simulink model "zoom_adc_single_pol"  (Simulink 7.8)
settings: Solver=FixedStepDiscrete  SolverMode=SingleTasking  StartTime=0.0  StopTime=4096  RelTol=1e-3
undefined symbols (not defined in the file): pfb_coeff_gen_calc
libraries: xbsIndex_r4 x413, casper_library_misc x48, xps_library x31, casper_library_delays x8, simulink x1
(part 1 of 6)
settings Model: Creator=jayanth  LastModifiedBy=dprice
settings Model: ModifiedComment=|
  | dprice -- Sun Apr 21 13:10:26 2013 -- Version 1.123
  | 
  | Added unsigned snap block to quant
settings Model: ModifiedHistory=|
  | dprice -- Sun Apr 21 13:10:26 2013 -- Version 1.123
  | 
  | Added unsigned snap block to quant
  | 
  | dprice -- Sun Apr 21 12:06:49 2013 -- Version 1.122
  | 
  | 
  | dprice -- Sun Apr 21 11:54:51 2013 -- Version 1.121
  | 
  | Changed over to quant block, added snap_quant for debugging
  | 
  | dprice -- Sun Apr 21 11:40:57 2013 -- Version 1.120
  | 
  | 
  | dprice -- Sun Apr 21 10:53:59 2013 -- Version 1.119
  | 
  | pkt_en going high now resets the packet counter in the header, and resets the 10 GbE core.
  | 
  | dprice -- Sat Apr 20 15:05:59 2013 -- Version 1.118
  | 
  | Fixed slice bug
  | 
  | dprice -- Sat Apr 20 14:12:55 2013 -- Version 1.117
  | 
  | Added a snap block after the quant
  | 
  | dprice -- Sat Apr 20 14:02:46 2013 -- Version 1.116
  | 
  | Trying to stop malformed packet being sent. Added in lots of pkt_en checks, so data is only valid when pkt_en is high
  | 
  | dprice -- Fri Apr 19 10:47:57 2013 -- Version 1.115
  | 
  | Switching to black boxed fft
settings DebuggingCC: FcnCallInpInsideContextMsg=Use local settings

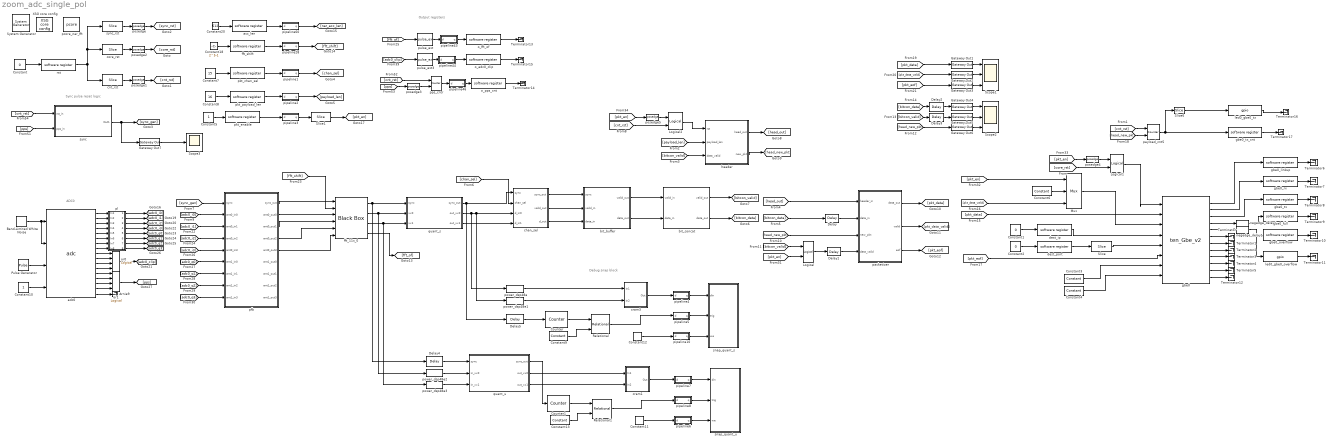
== system zoom_adc_single_pol ==
  note: Sync pulse reset logic
  note: ADC0
  note: Output registers
  note: Debug snap block
  " System Generator" : xbsIndex_r4/ System Generator  Tag=genX  xilinxfamily=virtex5  part=xc5vsx95t  speed=-1  package=ff1136  synthesis_tool=XST  clock_wrapper=Clock Enables  directory=./zoom_adc_single_pol/sysgen  proj_type=Project Navigator  Synth_file=XST Defaults  Impl_file=ISE Defaults  testbench=off  simulink_period=1  sysclk_period=5  dcm_input_clock_period=100  incr_netlist=off  trim_vbits=Everywhere in SubSystem  dbl_ovrd=According to Block Masks  core_generation=According to Block Masks  run_coregen=off  deprecated_control=off  eval_field=0  block_type=sysgen
  Arnie9 : Terminator
  Band-Limited White Noise : simulink/Sources/Band-Limited White Noise  Cov=[0.1]  Ts=0.1  seed=[23341]
  Constant : Constant  Value=0
  Constant1 : Constant  Value=0
  Constant10 : Constant
  Constant11 : xbsIndex_r4/Constant  const=1  gui_display_data_type=Boolean  arith_type=Boolean  n_bits=32  bin_pt=0  preci_type=Single  exp_width=8  frac_width=24  explicit_period=on  period=1  equ=P=C  opselect=C  inp2=PCIN>>17  opr=+  inp1=P  carry=CIN  dbl_ovrd=off  block_type=constant
  Constant12 : xbsIndex_r4/Constant  const=1  gui_display_data_type=Boolean  arith_type=Boolean  n_bits=32  bin_pt=0  preci_type=Single  exp_width=8  frac_width=24  explicit_period=on  period=1  equ=P=C  opselect=C  inp2=PCIN>>17  opr=+  inp1=P  carry=CIN  dbl_ovrd=off  block_type=constant
  Constant13 : xbsIndex_r4/Constant  const=0  gui_display_data_type=Fixed-point  arith_type=Signed (2's comp)  n_bits=3  bin_pt=0  preci_type=Single  exp_width=8  frac_width=24  explicit_period=on  period=1  equ=P=C  opselect=C  inp2=PCIN>>17  opr=+  inp1=P  carry=CIN  dbl_ovrd=off  block_type=constant
  Constant18 : Constant  Value=2^5-1
  Constant2 : Constant  Value=0
  Constant20 : Constant  Value=512
  Constant3 : xbsIndex_r4/Constant  const=1  gui_display_data_type=Boolean  arith_type=Boolean  n_bits=16  bin_pt=14  preci_type=Single  exp_width=8  frac_width=24  explicit_period=on  period=1  equ=P=C  opselect=C  inp2=PCIN>>17  opr=+  inp1=P  carry=CIN  dbl_ovrd=off  block_type=constant
  Constant4 : xbsIndex_r4/Constant  const=0  gui_display_data_type=Boolean  arith_type=Boolean  n_bits=16  bin_pt=14  preci_type=Single  exp_width=8  frac_width=24  explicit_period=on  period=1  equ=P=C  opselect=C  inp2=PCIN>>17  opr=+  inp1=P  carry=CIN  dbl_ovrd=off  block_type=constant
  Constant5 : Constant
  Constant6 : xbsIndex_r4/Constant  const=0  gui_display_data_type=Boolean  arith_type=Boolean  n_bits=16  bin_pt=14  preci_type=Single  exp_width=8  frac_width=24  explicit_period=off  period=1  equ=P=C  opselect=C  inp2=PCIN>>17  opr=+  inp1=P  carry=CIN  dbl_ovrd=off  block_type=constant
  Constant7 : Constant  Value=15
  Constant8 : Constant  Value=16
  Constant9 : xbsIndex_r4/Constant  const=0  gui_display_data_type=Fixed-point  arith_type=Signed (2's comp)  n_bits=3  bin_pt=0  preci_type=Single  exp_width=8  frac_width=24  explicit_period=on  period=1  equ=P=C  opselect=C  inp2=PCIN>>17  opr=+  inp1=P  carry=CIN  dbl_ovrd=off  block_type=constant
  Counter : xbsIndex_r4/Counter  cnt_type=Free Running  cnt_to=Inf  operation=Up  start_count=0  cnt_by_val=1  arith_type=Unsigned  n_bits=3  bin_pt=0  load_pin=off  rst=on  en=off  explicit_period=on  period=1  dbl_ovrd=off  use_behavioral_HDL=off  implementation=Fabric  block_type=counter
  Counter1 : xbsIndex_r4/Counter  cnt_type=Free Running  cnt_to=Inf  operation=Up  start_count=0  cnt_by_val=1  arith_type=Unsigned  n_bits=3  bin_pt=0  load_pin=off  rst=on  en=off  explicit_period=on  period=1  dbl_ovrd=off  use_behavioral_HDL=off  implementation=Fabric  block_type=counter
  Delay{,1..3} (4 alike) : xbsIndex_r4/Delay  rst=off  infoeditControl=Selection of Reset will increase slice count due to use of real FFs and instead of SRLs  en=off  latency=1  dbl_ovrd=off  reg_retiming=off  block_type=delay
  Delay4 : xbsIndex_r4/Delay  rst=off  infoeditControl=Selection of Reset will increase slice count due to use of real FFs and instead of SRLs  en=off  latency=4  dbl_ovrd=off  reg_retiming=off  block_type=delay
  Delay5 : xbsIndex_r4/Delay  rst=off  infoeditControl=Selection of Reset will increase slice count due to use of real FFs and instead of SRLs  en=off  latency=4  dbl_ovrd=off  reg_retiming=off  block_type=delay
  Gateway Out{1..7} (7 alike) : xbsIndex_r4/Gateway Out  inherit_from_input=off  hdl_port=on  timing_constraint=None  locs_specified=off  LOCs={}  UseAsDAC=off  DACChannel='1'  block_type=gatewayout
      settings: infoedit="Gateway out block.  Converts Xilinx fixed-point or floating-point type inputs into ouputs of type Simulink integer, single, double, or fixed point.<br><br>Hardware notes:  In hardware these blocks become top level output ports or are discarded, depending on how they are configured."
  Logical : xbsIndex_r4/Logical  logical_function=AND  inputs=2  en=off  latency=0  precision=Full  arith_type=Unsigned  n_bits=16  bin_pt=0  align_bp=on  dbl_ovrd=off  block_type=logical
  Logical1 : xbsIndex_r4/Logical  logical_function=OR  inputs=2  en=off  latency=0  precision=Full  arith_type=Unsigned  n_bits=16  bin_pt=0  align_bp=on  dbl_ovrd=off  block_type=logical
  Logical2 : xbsIndex_r4/Logical  logical_function=OR  inputs=2  en=off  latency=0  precision=Full  arith_type=Unsigned  n_bits=16  bin_pt=0  align_bp=on  dbl_ovrd=off  block_type=logical
  Mux : xbsIndex_r4/Mux  inputs=2  en=off  latency=0  precision=Full  arith_type=Unsigned  n_bits=16  bin_pt=14  quantization=Truncate  overflow=Wrap  dbl_ovrd=off  block_type=mux
  Pulse Generator : DiscretePulseGenerator  PulseType=Time based  Period=10  PulseWidth=5
  Relational : xbsIndex_r4/Relational  mode=a=b  en=off  latency=0  dbl_ovrd=off  block_type=relational
  Relational1 : xbsIndex_r4/Relational  mode=a=b  en=off  latency=0  dbl_ovrd=off  block_type=relational
  Scope1 : Scope  NumInputPorts=3
      settings: TimeRange=290.1459854014598  YMin=9.44473e+21~0~-1  YMax=3.5e+38~1~1
  Scope2 : Scope  NumInputPorts=3
      settings: TimeRange=290.1459854014598  YMin=0~0~0  YMax=1.2e+18~1~1
  Scope3 : Scope
      settings: SaveName=ScopeData6
  Slice : xbsIndex_r4/Slice  nbits=16  boolean_output=off  mode=Lower Bit Location + Width  bit1=0  base1=MSB of Input  bit0=0  base0=LSB of Input  dbl_ovrd=off  block_type=slice
  Slice1 : xbsIndex_r4/Slice  nbits=1  boolean_output=on  mode=Lower Bit Location + Width  bit1=1  base1=MSB of Input  bit0=0  base0=LSB of Input  dbl_ovrd=off  block_type=slice
      settings: block_version=10.1.3
  Slice6 : xbsIndex_r4/Slice  nbits=1  boolean_output=on  mode=Lower Bit Location + Width  bit1=0  base1=MSB of Input  bit0=15  base0=LSB of Input  dbl_ovrd=off  block_type=slice
      settings: block_version=10.1.3
  Terminator{,1..17} (18 alike) : Terminator
  XSG core config : xps_library/XSG core config  Tag=xps:xsg  hw_sys=ROACH:sx95t  ibob_linux=off  clk_src=adc0_clk  iBOB_clk_src=sys_clk  BEE2_ctrl_clk_src=sys_clk  BEE2_usr_clk_src=sys_clk  ROACH_clk_src=adc0_clk  ROACH2_clk_src=adc0_clk  CORR_clk_src=sys_clk  gpio_clk_io_group=iBOB:sma  gpio_clk_bit_index=0  clk_rate=200  sample_period=1  synthesis_tool=XST  mpc_type=powerpc440_ext
  acc_len : xps_library/software register  Tag=xps:sw_reg  io_dir=From Processor  arith_type=Unsigned  bitwidth=32  bin_pt=0  sample_period=1  gw_name=zoom_adc_single_pol_acc_len_user_data_out
      link override coarse_r01_acc_len_user_data_out: arith_type=Unsigned  n_bits=32  bin_pt=0  period=1
      link override coarse_r02_acc_len_user_data_out: arith_type=Unsigned  n_bits=32  bin_pt=0  period=1
      link override coarse_r03_acc_len_user_data_out: arith_type=Unsigned  n_bits=32  bin_pt=0  period=1
      link override coarse_r04_acc_len_user_data_out: arith_type=Unsigned  n_bits=32  bin_pt=0  period=1
      link override coarse_r06_acc_len_user_data_out: arith_type=Unsigned  n_bits=32  bin_pt=0  period=1
      link override coarse_r07_acc_len_user_data_out: arith_type=Unsigned  n_bits=32  bin_pt=0  period=1
      link override coarse_r08_acc_len_user_data_out: arith_type=Unsigned  n_bits=32  bin_pt=0  period=1
      link override coarse_r09_acc_len_user_data_out: arith_type=Unsigned  n_bits=32  bin_pt=0  period=1
      link override coarse_r10_acc_len_user_data_out: arith_type=Unsigned  n_bits=32  bin_pt=0  period=1
      link override coarse_r12_acc_len_user_data_out: arith_type=Unsigned  n_bits=32  bin_pt=0  period=1
      link override convert: arith_type=Unsigned  n_bits=32  bin_pt=0
      link override qdr_single_r01_acc_len_coarse_user_data_out: arith_type=Unsigned  n_bits=32  bin_pt=0  period=1
      link override qdr_single_r02_acc_len_coarse_user_data_out: arith_type=Unsigned  n_bits=32  bin_pt=0  period=1
      link override qdr_single_r04_acc_len_coarse_user_data_out: arith_type=Unsigned  n_bits=32  bin_pt=0  period=1
      link override r_spec_2048_r102_acc_len_user_data_out: arith_type=Unsigned  n_bits=32  bin_pt=0  period=1
      link override r_spec_2048_r102_nosim_acc_len_user_data_out: arith_type=Unsigned  n_bits=32  bin_pt=0  period=1
      link override r_spec_2048_r103_acc_len_user_data_out: arith_type=Unsigned  n_bits=32  bin_pt=0  period=1
      link override r_spec_2048_r104_acc_len_user_data_out: arith_type=Unsigned  n_bits=32  bin_pt=0  period=1
      link override r_spec_2048_r104_test0_acc_len_user_data_out: arith_type=Unsigned  n_bits=32  bin_pt=0  period=1
      link override r_spec_2048_r104_test_acc_len_user_data_out: arith_type=Unsigned  n_bits=32  bin_pt=0  period=1
      link override r_spec_2048_r105_acc_len_user_data_out: arith_type=Unsigned  n_bits=32  bin_pt=0  period=1
      link override r_spec_test0_acc_len_user_data_out: arith_type=Unsigned  n_bits=32  bin_pt=0  period=1
      link override r_spec_test4_acc_len_user_data_out: arith_type=Unsigned  n_bits=32  bin_pt=0  period=1
      link override roach_spec_acc_len_user_data_out: arith_type=Unsigned  n_bits=32  bin_pt=0  period=1
      link override roach_spec_no10gbe_acc_len_user_data_out: arith_type=Unsigned  n_bits=32  bin_pt=0  period=1
      link override roach_spec_rst_sync_cnt_user_data_out: arith_type=Unsigned  n_bits=32  bin_pt=0  period=1
      link override toast_256ch_16bit_r02_acc_len_user_data_out: arith_type=Unsigned  n_bits=32  bin_pt=0  period=1
      link override toast_256ch_16bit_r04_acc_len_user_data_out: arith_type=Unsigned  n_bits=32  bin_pt=0  period=1
      link override toast_256ch_16bit_r05_acc_len_user_data_out: arith_type=Unsigned  n_bits=32  bin_pt=0  period=1
  adc0 : xps_library/adc  Tag=xps:adc  adc_brd=adc0  adc_clk_rate=800  adc_interleave=off  sample_period=1
  bit_buffer : Subsystem
  bit_concat : Subsystem
  chan_sel : Subsystem
  cnt_rst : xbsIndex_r4/Slice  nbits=1  boolean_output=on  mode=Lower Bit Location + Width  bit1=0  base1=MSB of Input  bit0=0  base0=LSB of Input  dbl_ovrd=off  block_type=slice
  core_rst : xbsIndex_r4/Slice  nbits=1  boolean_output=on  mode=Lower Bit Location + Width  bit1=0  base1=MSB of Input  bit0=1  base0=LSB of Input  dbl_ovrd=off  block_type=slice
  cram1 : Subsystem  AncestorBlock=gavrt_library/cram  mask(cram){num_slice=2}
      mask prompts: num_slice "Number of slices"
      mask help: Concatenates inputs together after forcing binary point to zero.
      mask init:
      | cram_init(gcb, ...
      |     'num_slice', num_slice);
  cram3 : Subsystem  AncestorBlock=gavrt_library/cram  mask(cram){num_slice=2}
      mask prompts: num_slice "Number of slices"
      mask help: Concatenates inputs together after forcing binary point to zero.
      mask init:
      | cram_init(gcb, ...
      |     'num_slice', num_slice);
  dest_ip : xps_library/software register  Tag=xps:sw_reg  io_dir=From Processor  arith_type=Unsigned  bitwidth=32  bin_pt=0  sample_period=1  gw_name=zoom_adc_single_pol_dest_ip_user_data_out
      link override hipsr_tgbe3_dest_ip_user_data_out: arith_type=Unsigned  n_bits=32  bin_pt=0  period=1
  dest_port : xps_library/software register  Tag=xps:sw_reg  io_dir=From Processor  arith_type=Unsigned  bitwidth=32  bin_pt=0  sample_period=1  gw_name=zoom_adc_single_pol_dest_port_user_data_out
      link override hipsr_tgbe3_dest_port_user_data_out: arith_type=Unsigned  n_bits=32  bin_pt=0  period=1
  fft_11x_0 : xbsIndex_r4/Black Box  init_code=fft_32pt_11x_core_config  sim_method=Inactive  verbose=off  block_type=blackbox2
  fft_shift : xps_library/software register  Tag=xps:sw_reg  io_dir=From Processor  arith_type=Unsigned  bitwidth=32  bin_pt=0  sample_period=1  gw_name=zoom_adc_single_pol_fft_shift_user_data_out
      link override coarse_r01_acc_len_user_data_out: arith_type=Unsigned  n_bits=32  bin_pt=0  period=1
      link override coarse_r02_acc_len_user_data_out: arith_type=Unsigned  n_bits=32  bin_pt=0  period=1
      link override coarse_r03_acc_len_user_data_out: arith_type=Unsigned  n_bits=32  bin_pt=0  period=1
      link override coarse_r04_acc_len_user_data_out: arith_type=Unsigned  n_bits=32  bin_pt=0  period=1
      link override coarse_r06_acc_len_user_data_out: arith_type=Unsigned  n_bits=32  bin_pt=0  period=1
      link override coarse_r07_acc_len_user_data_out: arith_type=Unsigned  n_bits=32  bin_pt=0  period=1
      link override coarse_r08_acc_len_user_data_out: arith_type=Unsigned  n_bits=32  bin_pt=0  period=1
      link override coarse_r09_acc_len_user_data_out: arith_type=Unsigned  n_bits=32  bin_pt=0  period=1
      link override coarse_r10_acc_len_user_data_out: arith_type=Unsigned  n_bits=32  bin_pt=0  period=1
      link override coarse_r12_acc_len_user_data_out: arith_type=Unsigned  n_bits=32  bin_pt=0  period=1
      link override convert: arith_type=Unsigned  n_bits=32  bin_pt=0
      link override qdr_single_r01_acc_len_coarse_user_data_out: arith_type=Unsigned  n_bits=32  bin_pt=0  period=1
      link override qdr_single_r02_acc_len_coarse_user_data_out: arith_type=Unsigned  n_bits=32  bin_pt=0  period=1
      link override qdr_single_r04_acc_len_coarse_user_data_out: arith_type=Unsigned  n_bits=32  bin_pt=0  period=1
      link override r_spec_2048_r102_acc_len_user_data_out: arith_type=Unsigned  n_bits=32  bin_pt=0  period=1
      link override r_spec_2048_r102_nosim_acc_len_user_data_out: arith_type=Unsigned  n_bits=32  bin_pt=0  period=1
      link override r_spec_2048_r103_acc_len_user_data_out: arith_type=Unsigned  n_bits=32  bin_pt=0  period=1
      link override r_spec_2048_r104_acc_len_user_data_out: arith_type=Unsigned  n_bits=32  bin_pt=0  period=1
      link override r_spec_2048_r104_test0_acc_len_user_data_out: arith_type=Unsigned  n_bits=32  bin_pt=0  period=1
      link override r_spec_2048_r104_test_acc_len_user_data_out: arith_type=Unsigned  n_bits=32  bin_pt=0  period=1
      link override r_spec_2048_r105_acc_len_user_data_out: arith_type=Unsigned  n_bits=32  bin_pt=0  period=1
      link override r_spec_test0_acc_len_user_data_out: arith_type=Unsigned  n_bits=32  bin_pt=0  period=1
      link override r_spec_test4_acc_len_user_data_out: arith_type=Unsigned  n_bits=32  bin_pt=0  period=1
      link override roach_spec_acc_len_user_data_out: arith_type=Unsigned  n_bits=32  bin_pt=0  period=1
      link override roach_spec_no10gbe_acc_len_user_data_out: arith_type=Unsigned  n_bits=32  bin_pt=0  period=1
      link override roach_spec_rst_sync_cnt_user_data_out: arith_type=Unsigned  n_bits=32  bin_pt=0  period=1
      link override toast_256ch_16bit_r02_acc_len_user_data_out: arith_type=Unsigned  n_bits=32  bin_pt=0  period=1
      link override toast_256ch_16bit_r04_acc_len_user_data_out: arith_type=Unsigned  n_bits=32  bin_pt=0  period=1
      link override toast_256ch_16bit_r05_acc_len_user_data_out: arith_type=Unsigned  n_bits=32  bin_pt=0  period=1
  gbe0 : xps_library/ten_Gbe_v2  Tag=xps:tengbe_v2  port=0  rx_dist_ram=off  large_frames=on  show_param=off  pre_emph=3  swing=800  fab_en=on  fab_mac=hex2dec('123456780000')  fab_ip=192*(2^24) + 168*(2^16) + 5*(2^8) + 20*(2^0)  fab_udp=10000  fab_gate=1  cpu_rx_en=on  cpu_tx_en=on
  gbe0_full : xps_library/software register  Tag=xps:sw_reg  io_dir=To Processor  arith_type=Unsigned  bitwidth=32  bin_pt=0  sample_period=1  gw_name=zoom_adc_single_pol_gbe0_full_user_data_in
      link override convert: arith_type=Unsigned  n_bits=32  bin_pt=0
  gbe0_linkup : xps_library/software register  Tag=xps:sw_reg  io_dir=To Processor  arith_type=Unsigned  bitwidth=32  bin_pt=0  sample_period=1  gw_name=zoom_adc_single_pol_gbe0_linkup_user_data_in
      link override convert: arith_type=Unsigned  n_bits=32  bin_pt=0
  gbe0_overflow : xps_library/software register  Tag=xps:sw_reg  io_dir=To Processor  arith_type=Unsigned  bitwidth=32  bin_pt=0  sample_period=1  gw_name=zoom_adc_single_pol_gbe0_overflow_user_data_in
      link override convert: arith_type=Unsigned  n_bits=32  bin_pt=0
  gbe0_rx : xps_library/software register  Tag=xps:sw_reg  io_dir=To Processor  arith_type=Unsigned  bitwidth=32  bin_pt=0  sample_period=1  gw_name=zoom_adc_single_pol_gbe0_rx_user_data_in
      link override convert: arith_type=Unsigned  n_bits=32  bin_pt=0
  gbe0_tx : xps_library/software register  Tag=xps:sw_reg  io_dir=To Processor  arith_type=Unsigned  bitwidth=32  bin_pt=0  sample_period=1  gw_name=zoom_adc_single_pol_gbe0_tx_user_data_in
      link override convert: arith_type=Unsigned  n_bits=32  bin_pt=0
  gbe0_tx_cnt : xps_library/software register  Tag=xps:sw_reg  io_dir=To Processor  arith_type=Unsigned  bitwidth=32  bin_pt=0  sample_period=1  gw_name=zoom_adc_single_pol_gbe0_tx_cnt_user_data_in
      link override convert: arith_type=Unsigned  n_bits=32  bin_pt=0
  header : Subsystem
  led0_gbe0_overflow : xps_library/gpio  Tag=xps:gpio  io_group=ROACH:led  io_dir=out  arith_type=Boolean  bitwidth=1  bin_pt=0  bit_index=1  sample_period=1  use_single_ended=off  use_ddr=off  reg_iob=on  reg_clk_phase=0  termination=None
      link override convert: arith_type=Boolean  n_bits=1  bin_pt=0
  led0_gbe0_tx : xps_library/gpio  Tag=xps:gpio  io_group=ROACH:led  io_dir=out  arith_type=Boolean  bitwidth=1  bin_pt=0  bit_index=0  sample_period=1  use_single_ended=off  use_ddr=off  reg_iob=off  reg_clk_phase=0  termination=None
      link override convert: arith_type=Boolean  n_bits=1  bin_pt=0
  negedge_delay : casper_library_misc/negedge_delay  pulse_len=2^20
  negedge_delay1 : casper_library_misc/negedge_delay  pulse_len=2^20
  o_adc0_clip : xps_library/software register  Tag=xps:sw_reg  io_dir=To Processor  arith_type=Unsigned  bitwidth=32  bin_pt=0  sample_period=1  gw_name=zoom_adc_single_pol_o_adc0_clip_user_data_in
      link override convert: arith_type=Unsigned  n_bits=32  bin_pt=0
  o_fft_of : xps_library/software register  Tag=xps:sw_reg  io_dir=To Processor  arith_type=Unsigned  bitwidth=32  bin_pt=0  sample_period=1  gw_name=zoom_adc_single_pol_o_fft_of_user_data_in
      link override convert: arith_type=Unsigned  n_bits=32  bin_pt=0
  o_pps_cnt : xps_library/software register  Tag=xps:sw_reg  io_dir=To Processor  arith_type=Unsigned  bitwidth=32  bin_pt=0  sample_period=1  gw_name=zoom_adc_single_pol_o_pps_cnt_user_data_in
      link override convert: arith_type=Unsigned  n_bits=32  bin_pt=0
  or0 : xbsIndex_r4/Logical  logical_function=OR  inputs=4  en=off  latency=2  precision=Full  arith_type=Unsigned  n_bits=16  bin_pt=0  align_bp=off  dbl_ovrd=off  block_type=logical
  or1 : xbsIndex_r4/Logical  logical_function=OR  inputs=4  en=off  latency=2  precision=Full  arith_type=Unsigned  n_bits=16  bin_pt=0  align_bp=off  dbl_ovrd=off  block_type=logical
  packetizer : Subsystem
  payload_cnt5 : xbsIndex_r4/Counter  cnt_type=Free Running  cnt_to=0  operation=Up  start_count=0  cnt_by_val=1  arith_type=Unsigned  n_bits=32  bin_pt=0  load_pin=off  rst=on  en=on  explicit_period=on  period=1  dbl_ovrd=off  use_behavioral_HDL=off  implementation=Fabric  use_rpm=on  block_type=counter
      settings: xl_area=[0, 0, 0, 0, 0, 0, 0]
  pcore_nar_fft : xps_library/pcore  Tag=xps:pcore  pcore_path=./bb/fft_32pt_11x_core/fft_32pt_11x_core.ngc
  pfb : Subsystem
  pipeline1 : Subsystem  AncestorBlock=casper_library_delays/pipeline  mask(pipeline){latency=1}
      mask help:
      | An explicitly laid-out delay line to avoid mapping to SRL16s
      | for use in pipelining to help achieve timing closure.
      mask init:
      | pipeline_init(gcb,'latency',latency);
      settings: AttributesFormatString=Latency = %<latency>
      mask Display:
      | port_label('input', 1, 'd');
      | port_label('output', 1, 'q');
      | disp(['Z^-', num2str(latency)]);
  pipeline10 : Subsystem  AncestorBlock=casper_library_delays/pipeline  mask(pipeline){latency=1}
      mask help:
      | An explicitly laid-out delay line to avoid mapping to SRL16s
      | for use in pipelining to help achieve timing closure.
      mask init:
      | pipeline_init(gcb,'latency',latency);
      settings: AttributesFormatString=Latency = %<latency>
      mask Display:
      | port_label('input', 1, 'd');
      | port_label('output', 1, 'q');
      | disp(['Z^-', num2str(latency)]);
  pipeline2 : Subsystem  AncestorBlock=casper_library_delays/pipeline  mask(pipeline){latency=1}
      mask help:
      | An explicitly laid-out delay line to avoid mapping to SRL16s
      | for use in pipelining to help achieve timing closure.
      mask init:
      | pipeline_init(gcb,'latency',latency);
      settings: AttributesFormatString=Latency = %<latency>
      mask Display:
      | port_label('input', 1, 'd');
      | port_label('output', 1, 'q');
      | disp(['Z^-', num2str(latency)]);
  pipeline28 : Subsystem  AncestorBlock=casper_library_delays/pipeline  mask(pipeline){latency=1}
      mask help:
      | An explicitly laid-out delay line to avoid mapping to SRL16s
      | for use in pipelining to help achieve timing closure.
      mask init:
      | pipeline_init(gcb,'latency',latency);
      settings: AttributesFormatString=Latency = %<latency>
      mask Display:
      | port_label('input', 1, 'd');
      | port_label('output', 1, 'q');
      | disp(['Z^-', num2str(latency)]);
  pipeline3 : Subsystem  AncestorBlock=casper_library_delays/pipeline  mask(pipeline){latency=1}
      mask help:
      | An explicitly laid-out delay line to avoid mapping to SRL16s
      | for use in pipelining to help achieve timing closure.
      mask init:
      | pipeline_init(gcb,'latency',latency);
      settings: AttributesFormatString=Latency = %<latency>
      mask Display:
      | port_label('input', 1, 'd');
      | port_label('output', 1, 'q');
      | disp(['Z^-', num2str(latency)]);
  pipeline4 : Subsystem  AncestorBlock=casper_library_delays/pipeline  mask(pipeline){latency=1}
      mask help:
      | An explicitly laid-out delay line to avoid mapping to SRL16s
      | for use in pipelining to help achieve timing closure.
      mask init:
      | pipeline_init(gcb,'latency',latency);
      settings: AttributesFormatString=Latency = %<latency>
      mask Display:
      | port_label('input', 1, 'd');
      | port_label('output', 1, 'q');
      | disp(['Z^-', num2str(latency)]);
  pipeline43 : Subsystem  AncestorBlock=casper_library_delays/pipeline  mask(pipeline){latency=1}
      mask help:
      | An explicitly laid-out delay line to avoid mapping to SRL16s
      | for use in pipelining to help achieve timing closure.
      mask init:
      | pipeline_init(gcb,'latency',latency);
      settings: AttributesFormatString=Latency = %<latency>
      mask Display:
      | port_label('input', 1, 'd');
      | port_label('output', 1, 'q');
      | disp(['Z^-', num2str(latency)]);
  pipeline44 : Subsystem  AncestorBlock=casper_library_delays/pipeline  mask(pipeline){latency=1}
      mask help:
      | An explicitly laid-out delay line to avoid mapping to SRL16s
      | for use in pipelining to help achieve timing closure.
      mask init:
      | pipeline_init(gcb,'latency',latency);
      settings: AttributesFormatString=Latency = %<latency>
      mask Display:
      | port_label('input', 1, 'd');
      | port_label('output', 1, 'q');
      | disp(['Z^-', num2str(latency)]);
  pipeline46 : Subsystem  AncestorBlock=casper_library_delays/pipeline  mask(pipeline){latency=1}
      mask help:
      | An explicitly laid-out delay line to avoid mapping to SRL16s
      | for use in pipelining to help achieve timing closure.
      mask init:
      | pipeline_init(gcb,'latency',latency);
      settings: AttributesFormatString=Latency = %<latency>
      mask Display:
      | port_label('input', 1, 'd');
      | port_label('output', 1, 'q');
      | disp(['Z^-', num2str(latency)]);
  pipeline5 : Subsystem  AncestorBlock=casper_library_delays/pipeline  mask(pipeline){latency=1}
      mask help:
      | An explicitly laid-out delay line to avoid mapping to SRL16s
      | for use in pipelining to help achieve timing closure.
      mask init:
      | pipeline_init(gcb,'latency',latency);
      settings: AttributesFormatString=Latency = %<latency>
      mask Display:
      | port_label('input', 1, 'd');
      | port_label('output', 1, 'q');
      | disp(['Z^-', num2str(latency)]);
  pipeline6 : Subsystem  AncestorBlock=casper_library_delays/pipeline  mask(pipeline){latency=1}
      mask help:
      | An explicitly laid-out delay line to avoid mapping to SRL16s
      | for use in pipelining to help achieve timing closure.
      mask init:
      | pipeline_init(gcb,'latency',latency);
      settings: AttributesFormatString=Latency = %<latency>
      mask Display:
      | port_label('input', 1, 'd');
      | port_label('output', 1, 'q');
      | disp(['Z^-', num2str(latency)]);
  pipeline60 : Subsystem  AncestorBlock=casper_library_delays/pipeline  mask(pipeline){latency=1}
      mask help:
      | An explicitly laid-out delay line to avoid mapping to SRL16s
      | for use in pipelining to help achieve timing closure.
      mask init:
      | pipeline_init(gcb,'latency',latency);
      settings: AttributesFormatString=Latency = %<latency>
      mask Display:
      | port_label('input', 1, 'd');
      | port_label('output', 1, 'q');
      | disp(['Z^-', num2str(latency)]);
  pipeline7 : Subsystem  AncestorBlock=casper_library_delays/pipeline  mask(pipeline){latency=1}
      mask help:
      | An explicitly laid-out delay line to avoid mapping to SRL16s
      | for use in pipelining to help achieve timing closure.
      mask init:
      | pipeline_init(gcb,'latency',latency);
      settings: AttributesFormatString=Latency = %<latency>
      mask Display:
      | port_label('input', 1, 'd');
      | port_label('output', 1, 'q');
      | disp(['Z^-', num2str(latency)]);
  pipeline8 : Subsystem  AncestorBlock=casper_library_delays/pipeline  mask(pipeline){latency=1}
      mask help:
      | An explicitly laid-out delay line to avoid mapping to SRL16s
      | for use in pipelining to help achieve timing closure.
      mask init:
      | pipeline_init(gcb,'latency',latency);
      settings: AttributesFormatString=Latency = %<latency>
      mask Display:
      | port_label('input', 1, 'd');
      | port_label('output', 1, 'q');
      | disp(['Z^-', num2str(latency)]);
  pkt_chan_sel : xps_library/software register  Tag=xps:sw_reg  io_dir=From Processor  arith_type=Unsigned  bitwidth=32  bin_pt=0  sample_period=1  gw_name=zoom_adc_single_pol_pkt_chan_sel_user_data_out
      link override hipsr_tgbe3_pkt_chan_sel_user_data_out: arith_type=Unsigned  n_bits=32  bin_pt=0  period=1
  pkt_enable : xps_library/software register  Tag=xps:sw_reg  io_dir=From Processor  arith_type=Unsigned  bitwidth=32  bin_pt=0  sample_period=1  gw_name=zoom_adc_single_pol_pkt_enable_user_data_out
      link override hipsr_tgbe3_pkt_enable_user_data_out: arith_type=Unsigned  n_bits=32  bin_pt=0  period=1
  pkt_payload_len : xps_library/software register  Tag=xps:sw_reg  io_dir=From Processor  arith_type=Unsigned  bitwidth=32  bin_pt=0  sample_period=1  gw_name=zoom_adc_single_pol_pkt_payload_len_user_data_out
      link override hipsr_tgbe3_pkt_payload_len_user_data_out: arith_type=Unsigned  n_bits=32  bin_pt=0  period=1
  pl : Subsystem
  posedge{,1..5} (6 alike) : casper_library_misc/posedge  Tag=Rising Edge Detector
  power_dsp48e : casper_library_misc/power_dsp48e  bitwidth=8
      link override slice_imag: nbits=bitwidth  boolean_output=off  mode=Lower Bit Location + Width  bit1=0  base1=MSB of Input  bit0=0  base0=LSB of Input  dbl_ovrd=off
      link override slice_real: nbits=bitwidth  boolean_output=off  mode=Upper Bit Location + Width  bit1=0  base1=MSB of Input  bit0=0  base0=LSB of Input  dbl_ovrd=off
      link override slice_imag: infoedit="Extracts a given range of bits from each input sample and presents it at the output.  The output type is ordinarily unsigned with binary point at zero, but can be Boolean when the slice is one bit wide.<br><br>Hardware notes: In hardware this block costs nothing."
      link override slice_real: infoedit="Extracts a given range of bits from each input sample and presents it at the output.  The output type is ordinarily unsigned with binary point at zero, but can be Boolean when the slice is one bit wide.<br><br>Hardware notes: In hardware this block costs nothing."
  power_dsp48e1 : casper_library_misc/power_dsp48e  bitwidth=8
      link override slice_imag: nbits=bitwidth  boolean_output=off  mode=Lower Bit Location + Width  bit1=0  base1=MSB of Input  bit0=0  base0=LSB of Input  dbl_ovrd=off
      link override slice_real: nbits=bitwidth  boolean_output=off  mode=Upper Bit Location + Width  bit1=0  base1=MSB of Input  bit0=0  base0=LSB of Input  dbl_ovrd=off
      link override slice_imag: infoedit="Extracts a given range of bits from each input sample and presents it at the output.  The output type is ordinarily unsigned with binary point at zero, but can be Boolean when the slice is one bit wide.<br><br>Hardware notes: In hardware this block costs nothing."
      link override slice_real: infoedit="Extracts a given range of bits from each input sample and presents it at the output.  The output type is ordinarily unsigned with binary point at zero, but can be Boolean when the slice is one bit wide.<br><br>Hardware notes: In hardware this block costs nothing."
  power_dsp48e2 : casper_library_misc/power_dsp48e  bitwidth=18
      link override slice_imag: nbits=bitwidth  boolean_output=off  mode=Lower Bit Location + Width  bit1=0  base1=MSB of Input  bit0=0  base0=LSB of Input  dbl_ovrd=off
      link override slice_real: nbits=bitwidth  boolean_output=off  mode=Upper Bit Location + Width  bit1=0  base1=MSB of Input  bit0=0  base0=LSB of Input  dbl_ovrd=off
      link override slice_imag: infoedit="Extracts a given range of bits from each input sample and presents it at the output.  The output type is ordinarily unsigned with binary point at zero, but can be Boolean when the slice is one bit wide.<br><br>Hardware notes: In hardware this block costs nothing."
      link override slice_real: infoedit="Extracts a given range of bits from each input sample and presents it at the output.  The output type is ordinarily unsigned with binary point at zero, but can be Boolean when the slice is one bit wide.<br><br>Hardware notes: In hardware this block costs nothing."
  power_dsp48e3 : casper_library_misc/power_dsp48e  bitwidth=18
      link override slice_imag: nbits=bitwidth  boolean_output=off  mode=Lower Bit Location + Width  bit1=0  base1=MSB of Input  bit0=0  base0=LSB of Input  dbl_ovrd=off
      link override slice_real: nbits=bitwidth  boolean_output=off  mode=Upper Bit Location + Width  bit1=0  base1=MSB of Input  bit0=0  base0=LSB of Input  dbl_ovrd=off
      link override slice_imag: infoedit="Extracts a given range of bits from each input sample and presents it at the output.  The output type is ordinarily unsigned with binary point at zero, but can be Boolean when the slice is one bit wide.<br><br>Hardware notes: In hardware this block costs nothing."
      link override slice_real: infoedit="Extracts a given range of bits from each input sample and presents it at the output.  The output type is ordinarily unsigned with binary point at zero, but can be Boolean when the slice is one bit wide.<br><br>Hardware notes: In hardware this block costs nothing."
  pps_cntr : xbsIndex_r4/Counter  cnt_type=Free Running  cnt_to=Inf  operation=Up  start_count=0  cnt_by_val=1  arith_type=Unsigned  n_bits=16  bin_pt=0  load_pin=off  rst=on  en=on  explicit_period=on  period=1  dbl_ovrd=off  use_behavioral_HDL=off  implementation=Fabric  use_rpm=off  block_type=counter
  pulse_ext : casper_library_misc/pulse_ext  pulse_len=100000
  pulse_ext3 : casper_library_misc/pulse_ext  pulse_len=100000
  quant_s : Subsystem  mask{bits_in=36, bits_out=8, z_cast=3, z_mult=4, quantization=Round  (unbiased: +/- Inf)}
      mask prompts: bits_in "Input bitwidth"; bits_out "Output bitwidth"; z_cast "Convert latency"; z_mult "Multiply latency"; quantization "Quantization Behaviour"
      mask help:
      | Requantizes a signal down to a desired bit width.
      | Best used in conjunction with the Stokes block.
      | Note: in_xx and in_yy are treated as unsigned, xy are treated as signed.
      mask StyleString: edit,edit,edit,edit,popup(Truncate|Round  (unbiased: +/- Inf)|Round  (unbiased: Even Values))
  quant_u : Subsystem  AncestorBlock=hipsr_library/quant  mask{bits_in=36, bits_out=16, z_cast=3, z_mult=3, quantization=Round  (unbiased: +/- Inf)}
      mask prompts: bits_in "Input bitwidth"; bits_out "Output bitwidth"; z_cast "Convert latency"; z_mult "Multiply latency"; quantization "Quantization Behaviour"
      mask help:
      | Requantizes a signal down to a desired bit width.
      | Best used in conjunction with the Stokes block.
      | Note: in_xx and in_yy are treated as unsigned, xy are treated as signed.
      mask StyleString: edit,edit,edit,edit,popup(Truncate|Round  (unbiased: +/- Inf)|Round  (unbiased: Even Values))
  rst : xps_library/software register  Tag=xps:sw_reg  io_dir=From Processor  arith_type=Unsigned  bitwidth=32  bin_pt=0  sample_period=1  gw_name=zoom_adc_single_pol_rst_user_data_out
      link override hipsr_tgbe3_rst_user_data_out: arith_type=Unsigned  n_bits=32  bin_pt=0  period=1
  snap_quant_s : Subsystem  AncestorBlock=casper_library_scopes/snap  mask(snap){nsamples=10}
      mask prompts: nsamples "No. of samples(2^?)"
      mask help:
      | The <i>snap</i> block provides a packaged solution to capturing data from
      | the FPGA fabric and making it accessible from the CPU.  The block comes in
      | 2 flavors: <i>snap</i> (which captures to a 32 bit wide Shared BRAM), and
      | <i>snap64</i> (which captures to 2x32 bit wide Shared BRAMs to effect a
      | 64 bit capture).
      mask Help: eval('xlWeb(''http://casper.berkeley.edu/wiki/Snap'')')
  snap_quant_u : Subsystem  AncestorBlock=casper_library_scopes/snap  mask(snap){nsamples=10}
      mask prompts: nsamples "No. of samples(2^?)"
      mask help:
      | The <i>snap</i> block provides a packaged solution to capturing data from
      | the FPGA fabric and making it accessible from the CPU.  The block comes in
      | 2 flavors: <i>snap</i> (which captures to a 32 bit wide Shared BRAM), and
      | <i>snap64</i> (which captures to 2x32 bit wide Shared BRAMs to effect a
      | 64 bit capture).
      mask Help: eval('xlWeb(''http://casper.berkeley.edu/wiki/Snap'')')
  sync : Subsystem  AncestorBlock=hipsr_library/sync
  sync_rst : xbsIndex_r4/Slice  nbits=1  boolean_output=on  mode=Lower Bit Location + Width  bit1=0  base1=MSB of Input  bit0=2  base0=LSB of Input  dbl_ovrd=off  block_type=slice
  wires:
  Constant/1 -> rst/1
  rst/1 -> cnt_rst/1, core_rst/1, sync_rst/1
  core_rst/1 -> posedge2/1
  cnt_rst/1 -> posedge1/1
  Constant2/1 -> dest_port/1
  Constant1/1 -> dest_ip/1
  dest_ip/1 -> gbe0/4
  dest_port/1 -> Slice/1
  Slice/1 -> gbe0/5
  gbe0/6 -> Terminator/1
  gbe0/7 -> Terminator1/1
  gbe0/8 -> Terminator2/1
  gbe0/9 -> Terminator3/1
  gbe0/10 -> Terminator4/1
  gbe0/11 -> Terminator5/1
  Constant3/1 -> gbe0/7
  gbe0/1 -> gbe0_linkup/1
  gbe0/2 -> gbe0_rx/1
  gbe0/3 -> gbe0_tx/1
  gbe0/4 -> negedge_delay/1
  negedge_delay/1 -> gbe0_full/1
  gbe0/5 -> negedge_delay1/1
  negedge_delay1/1 -> gbe0_overflow/1, led0_gbe0_overflow/1
  payload_cnt5/1 -> Slice6/1, gbe0_tx_cnt/1
  Slice6/1 -> led0_gbe0_tx/1
  [cnt_rst] -> payload_cnt5/1
  led0_gbe0_tx/1 -> Terminator16/1
  gbe0_tx_cnt/1 -> Terminator17/1
  gbe0_linkup/1 -> Terminator6/1
  gbe0_rx/1 -> Terminator7/1
  gbe0_tx/1 -> Terminator8/1
  gbe0_full/1 -> Terminator9/1
  gbe0_overflow/1 -> Terminator10/1
  led0_gbe0_overflow/1 -> Terminator11/1
  Constant4/1 -> gbe0/8
  gbe0/12 -> Terminator12/1
  sync_rst/1 -> posedge/1
  posedge/1 -> [sync_rst]
  posedge1/1 -> [cnt_rst]
  posedge2/1 -> [core_rst]
  Constant7/1 -> pkt_chan_sel/1
  pkt_chan_sel/1 -> pipeline1/1(d)
  Gateway Out4/1 -> Scope2/1
  Gateway Out5/1 -> Scope2/2
  Gateway Out6/1 -> Scope2/3
  [pkt_en] -> Mux/1
  Constant6/1 -> Mux/2
  Mux/1 -> gbe0/3
  [pkt_data] -> gbe0/2
  Constant8/1 -> pkt_payload_len/1
  pkt_payload_len/1 -> pipeline2/1(d)
  bit_buffer/2(data_out) -> bit_concat/2(data_in)
  bit_concat/2(data_out) -> [bitcon_data]
  bit_concat/1(valid_out) -> [bitcon_valid]
  [payload_len] -> header/2(payload_len)
  [bitcon_valid] -> header/3(data_valid)
  header/1(head_out) -> [head_out]
  [head_out] -> packetizer/1(header_in)
  [bitcon_data] -> Delay/1
  header/2(new_pkt) -> [head_new_pkt]
  [head_new_pkt] -> packetizer/3(new_pkt)
  packetizer/1(data_out) -> [pkt_data]
  packetizer/2(valid) -> [pkt_data_valid]
  packetizer/3(eof) -> [pkt_eof]
  [bitcon_data] -> Delay2/1
  [bitcon_valid] -> Delay3/1
  [head_new_pkt] -> Gateway Out6/1
  [pkt_data_valid] -> Mux/3
  [pkt_eof] -> gbe0/6
  [head_new_pkt] -> payload_cnt5/2
  Gateway Out1/1 -> Scope1/1
  Gateway Out2/1 -> Scope1/2
  Gateway Out3/1 -> Scope1/3
  [pkt_data] -> Gateway Out1/1
  [pkt_data_valid] -> Gateway Out2/1
  [pkt_eof] -> Gateway Out3/1
  Delay/1 -> packetizer/2(data_in)
  Delay1/1 -> packetizer/4(data_valid)
  Delay2/1 -> Gateway Out4/1
  Delay3/1 -> Gateway Out5/1
  pfb/2(ant0_out0) -> fft_11x_0/3
  pfb/3(ant0_out1) -> fft_11x_0/4
  pfb/4(ant0_out2) -> fft_11x_0/5
  pfb/5(ant0_out3) -> fft_11x_0/6
  pfb/1(sync_out) -> fft_11x_0/1
  fft_11x_0/4 -> [fft_of]
  [fft_shift] -> fft_11x_0/2
  [pps] -> sync/2(pps_in)
  sync/1(Out1) -> [sync_gen], Gateway Out7/1
  [cnt_rst] -> sync/1(rst_in)
  Gateway Out7/1 -> Scope3/1
  Constant18/1 -> fft_shift/1
  fft_shift/1 -> pipeline28/1(d)
  pipeline28/1(q) -> [fft_shift]
  Constant20/1 -> acc_len/1
  acc_len/1 -> pipeline60/1(d)
  pipeline60/1(q) -> [nar_acc_len]
  [chan_sel] -> chan_sel/2(chan_sel)
  chan_sel/1(sync_out) -> bit_buffer/1(sync)
  chan_sel/2(valid_out) -> bit_buffer/2(valid_in)
  chan_sel/3(d_out) -> bit_buffer/3(data_in)
  [sync_gen] -> pfb/1(sync)
  Band-Limited White Noise/1 -> adc0/1, adc0/2
  Pulse Generator/1 -> adc0/3
  Constant10/1 -> adc0/4
  adc0/9 -> or0/1
  adc0/10 -> or0/2
  adc0/11 -> or0/3
  adc0/12 -> or0/4
  adc0/13 -> or1/1
  adc0/14 -> or1/2
  adc0/15 -> or1/3
  adc0/16 -> or1/4
  adc0/17 -> Arnie9/1
  or0/1 -> [adc0_clip]
  or1/1 -> [pps]
  adc0/1 -> pl/1(In1)
  adc0/2 -> pl/2(In2)
  adc0/3 -> pl/3(In3)
  adc0/4 -> pl/4(In4)
  adc0/5 -> pl/5(In5)
  adc0/6 -> pl/6(In6)
  adc0/7 -> pl/7(In7)
  adc0/8 -> pl/8(In8)
  pl/1(Out1) -> [adc0_i0]
  pl/2(Out2) -> [adc0_i1]
  pl/3(Out3) -> [adc0_i2]
  pl/4(Out4) -> [adc0_i3]
  pl/5(Out5) -> [adc0_q0]
  pl/6(Out6) -> [adc0_q1]
  pl/7(Out7) -> [adc0_q2]
  pl/8(Out8) -> [adc0_q3]
  [adc0_q3] -> pfb/9(ant1_in3)
  [adc0_q2] -> pfb/8(ant1_in2)
  [adc0_q1] -> pfb/7(ant1_in1)
  [adc0_q0] -> pfb/6(ant1_in0)
  [adc0_i3] -> pfb/5(ant0_in3)
  [adc0_i2] -> pfb/4(ant0_in2)
  [adc0_i1] -> pfb/3(ant0_in1)
  [adc0_i0] -> pfb/2(ant0_in0)
  pipeline43/1(q) -> o_fft_of/1
  o_fft_of/1 -> Terminator13/1
  pipeline44/1(q) -> o_adc0_clip/1
  [adc0_clip] -> pulse_ext3/1
  o_adc0_clip/1 -> Terminator15/1
  pulse_ext3/1 -> pipeline44/1(d)
  [fft_of] -> pulse_ext/1
  pulse_ext/1 -> pipeline43/1(d)
  pps_cntr/1 -> pipeline46/1(d)
  pipeline46/1(q) -> o_pps_cnt/1
  o_pps_cnt/1 -> Terminator14/1
  [cnt_rst] -> pps_cntr/1
  posedge3/1 -> pps_cntr/2
  [pps] -> posedge3/1
  pipeline1/1(q) -> [chan_sel]
  pipeline2/1(q) -> [payload_len]
  fft_11x_0/1 -> quant_s/1(sync), Delay4/1
  fft_11x_0/2 -> quant_s/2(xx0), power_dsp48e2/1
  fft_11x_0/3 -> quant_s/3(xx1), power_dsp48e3/1
  Constant5/1 -> pkt_enable/1
  pkt_enable/1 -> pipeline3/1(d)
  pipeline3/1(q) -> Slice1/1
  bit_buffer/1(valid_out) -> bit_concat/1(valid_in)
  [pkt_en] -> Logical/2
  [bitcon_valid] -> Logical/1
  Logical/1 -> Delay1/1
  Slice1/1 -> [pkt_en]
  [core_rst] -> Logical1/2
  [pkt_en] -> posedge4/1
  Logical1/1 -> gbe0/1
  posedge4/1 -> Logical1/1
  [pkt_en] -> posedge5/1
  posedge5/1 -> Logical2/1
  [cnt_rst] -> Logical2/2
  Logical2/1 -> header/1(rst)
  quant_s/1(sync_out) -> chan_sel/1(sync), Delay5/1
  quant_s/2(out_xx0) -> power_dsp48e/1, chan_sel/3(d_in0), power_dsp48e1/1
  quant_s/3(out_xx1) -> chan_sel/4(d_in1)
  pipeline4/1(q) -> snap_quant_s/1(din)
  pipeline5/1(q) -> snap_quant_s/2(trig)
  pipeline10/1(q) -> snap_quant_s/3(we)
  power_dsp48e/1 -> cram3/1(In1)
  power_dsp48e1/1 -> cram3/2(In2)
  cram3/1(Out) -> pipeline4/1(d)
  Constant12/1 -> pipeline10/1(d)
  Counter/1 -> Relational/1
  Constant9/1 -> Relational/2
  Relational/1 -> pipeline5/1(d)
  pipeline7/1(q) -> snap_quant_u/1(din)
  pipeline8/1(q) -> snap_quant_u/2(trig)
  pipeline6/1(q) -> snap_quant_u/3(we)
  quant_u/2(out_xx0) -> cram1/1(In1)
  quant_u/3(out_xx1) -> cram1/2(In2)
  cram1/1(Out) -> pipeline7/1(d)
  Constant11/1 -> pipeline6/1(d)
  Counter1/1 -> Relational1/1
  Constant13/1 -> Relational1/2
  Relational1/1 -> pipeline8/1(d)
  power_dsp48e2/1 -> quant_u/2(in_xx0)
  power_dsp48e3/1 -> quant_u/3(in_xx1)
  Delay4/1 -> quant_u/1(sync)
  quant_u/1(sync_out) -> Counter1/1
  Delay5/1 -> Counter/1

== system zoom_adc_single_pol/bit_buffer ==
  sync : Inport
  valid_in : Inport  Port=2
  data_in : Inport  Port=3
  FIFO : xbsIndex_r4/FIFO  performance_options=Standard_FIFO  depth=16  percent_nbits=1  rst=on  en=off  use_dcount=off  use_percent_full_port=off  use_almost_empty=off  almost_empty_thresh=2  use_almost_full=off  almost_full_thresh=14  dbl_ovrd=off  mem_type=Block RAM  explicit_period=off  block_type=fifo
  Gateway Out{,1..3} (4 alike) : xbsIndex_r4/Gateway Out  inherit_from_input=off  hdl_port=on  timing_constraint=None  locs_specified=off  LOCs={}  UseAsDAC=off  DACChannel='1'  block_type=gatewayout
      settings: infoedit="Gateway out block.  Converts Xilinx fixed-point or floating-point type inputs into ouputs of type Simulink integer, single, double, or fixed point.<br><br>Hardware notes:  In hardware these blocks become top level output ports or are discarded, depending on how they are configured."
  Scope1 : Scope  NumInputPorts=2
      settings: YMin=-5~-5  YMax=5~5  SaveName=ScopeData3
  Scope2 : Scope  NumInputPorts=2
      settings: YMin=-5~-5  YMax=5~5  SaveName=ScopeData2
  fifo_re : Subsystem  mask{buf_len=2}
      mask prompts: buf_len "Buffer length (2^N)"
      mask help:
      | Read enabler block for FIFO buffer. Counts for desired number of valid datum,
      | then spits out data in a chunk.
  valid_out : Outport
  data_out : Outport  Port=2
  wires:
  data_in/1 -> FIFO/1, Gateway Out2/1
  valid_in/1 -> fifo_re/2(valid_in), FIFO/2, Gateway Out3/1
  sync/1 -> FIFO/4, fifo_re/1(rst)
  FIFO/1 -> data_out/1, Gateway Out/1
  fifo_re/1(re_out) -> FIFO/3, valid_out/1, Gateway Out1/1
  Gateway Out/1 -> Scope1/1
  Gateway Out1/1 -> Scope1/2
  Gateway Out2/1 -> Scope2/1
  Gateway Out3/1 -> Scope2/2

== system zoom_adc_single_pol/bit_concat ==
  valid_in : Inport
  data_in : Inport  Port=2
  Delay : xbsIndex_r4/Delay  rst=off  infoeditControl=Selection of Reset will increase slice count due to use of real FFs and instead of SRLs  en=off  latency=7  dbl_ovrd=off  reg_retiming=off  block_type=delay
  Gateway Out{,1..3} (4 alike) : xbsIndex_r4/Gateway Out  inherit_from_input=off  hdl_port=on  timing_constraint=None  locs_specified=off  LOCs={}  UseAsDAC=off  DACChannel='1'  block_type=gatewayout
      settings: infoedit="Gateway out block.  Converts Xilinx fixed-point or floating-point type inputs into ouputs of type Simulink integer, single, double, or fixed point.<br><br>Hardware notes:  In hardware these blocks become top level output ports or are discarded, depending on how they are configured."
  Scope : Scope  NumInputPorts=4
      settings: YMin=-5~-5~-5~-5  YMax=5~5~5~5  SaveName=ScopeData7
  cram : Subsystem  AncestorBlock=gavrt_library/cram  mask(cram){num_slice=4}
      mask prompts: num_slice "Number of slices"
      mask help: Concatenates inputs together after forcing binary point to zero.
      mask init:
      | cram_init(gcb, ...
      |     'num_slice', num_slice);
  delay_line : Subsystem
  posedge : casper_library_misc/posedge  Tag=Rising Edge Detector
  valid_out : Outport
  data_out : Outport  Port=2
  wires:
  data_in/1 -> delay_line/1(In1)
  delay_line/1(o1) -> cram/1(In1), Gateway Out1/1
  delay_line/2(o2) -> cram/2(In2), Gateway Out2/1
  delay_line/3(o3) -> cram/3(In3), Gateway Out3/1
  delay_line/4(o4) -> cram/4(In4)
  valid_in/1 -> posedge/1
  posedge/1 -> Delay/1
  Delay/1 -> valid_out/1, Gateway Out/1
  cram/1(Out) -> data_out/1
  Gateway Out/1 -> Scope/1
  Gateway Out1/1 -> Scope/2
  Gateway Out2/1 -> Scope/3
  Gateway Out3/1 -> Scope/4

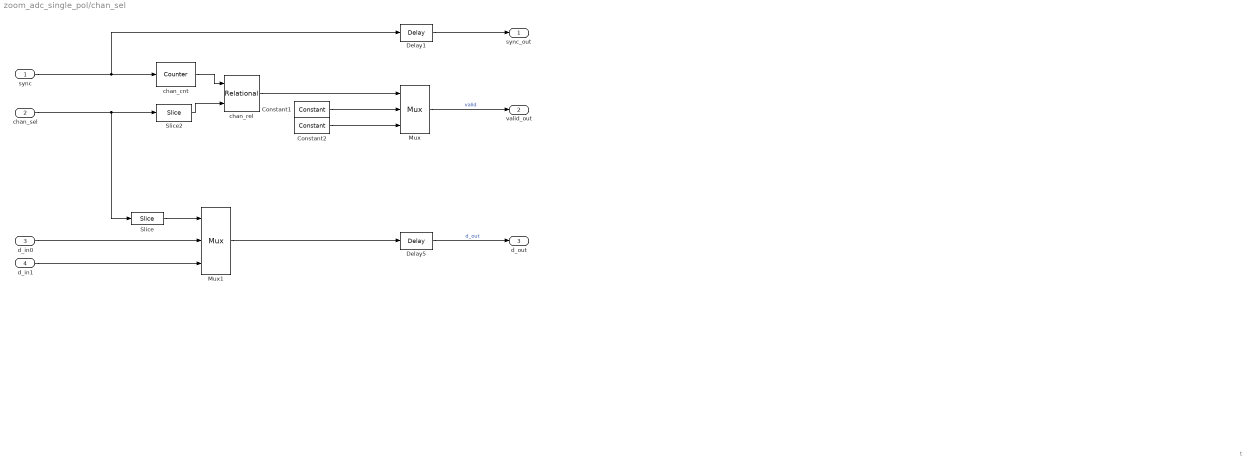
== system zoom_adc_single_pol/chan_sel ==
  note: t
  sync : Inport
  chan_sel : Inport  Port=2
  d_in0 : Inport  Port=3
  d_in1 : Inport  Port=4
  Constant1 : xbsIndex_r4/Constant  const=0  gui_display_data_type=Fixed-point  arith_type=Boolean  n_bits=1  bin_pt=0  preci_type=Single  exp_width=8  frac_width=24  explicit_period=on  period=1  equ=P=C  opselect=C  inp2=PCIN>>17  opr=+  inp1=P  carry=CIN  dbl_ovrd=off  block_type=constant
  Constant2 : xbsIndex_r4/Constant  const=1  gui_display_data_type=Boolean  arith_type=Boolean  n_bits=1  bin_pt=0  preci_type=Single  exp_width=8  frac_width=24  explicit_period=on  period=1  equ=P=C  opselect=C  inp2=PCIN>>17  opr=+  inp1=P  carry=CIN  dbl_ovrd=off  block_type=constant
  Delay1 : xbsIndex_r4/Delay  rst=off  infoeditControl=Selection of Reset will increase slice count due to use of real FFs and instead of SRLs  en=off  latency=1  dbl_ovrd=off  reg_retiming=on  block_type=delay
      settings: xl_area=[0, 0, 0, 0, 0, 0, 0]
  Delay5 : xbsIndex_r4/Delay  rst=off  infoeditControl=Selection of Reset will increase slice count due to use of real FFs and instead of SRLs  en=off  latency=1  dbl_ovrd=off  reg_retiming=on  block_type=delay
      settings: xl_area=[0, 0, 0, 0, 0, 0, 0]
  Mux : xbsIndex_r4/Mux  inputs=2  en=off  latency=1  precision=Full  arith_type="Signed  (2's comp)"  n_bits=8  bin_pt=2  quantization=Truncate  overflow=Wrap  dbl_ovrd=off  block_type=mux
      settings: xl_area=[0, 0, 0, 0, 0, 0, 0]
  Mux1 : xbsIndex_r4/Mux  inputs=2  en=off  latency=0  precision=Full  arith_type=Unsigned  n_bits=16  bin_pt=14  quantization=Truncate  overflow=Wrap  dbl_ovrd=off  block_type=mux
  Slice : xbsIndex_r4/Slice  nbits=1  boolean_output=off  mode=Lower Bit Location + Width  bit1=0  base1=MSB of Input  bit0=0  base0=LSB of Input  dbl_ovrd=off  block_type=slice
  Slice2 : xbsIndex_r4/Slice  nbits=4  boolean_output=off  mode=Lower Bit Location + Width  bit1=1  base1=MSB of Input  bit0=1  base0=LSB of Input  dbl_ovrd=off  block_type=slice
      settings: block_version=10.1.3
  chan_cnt : xbsIndex_r4/Counter  cnt_type=Free Running  cnt_to=Inf  operation=Up  start_count=0  cnt_by_val=1  arith_type=Unsigned  n_bits=4  bin_pt=0  load_pin=off  rst=on  en=off  explicit_period=on  period=1  dbl_ovrd=off  use_behavioral_HDL=off  implementation=Fabric  block_type=counter
  chan_rel : xbsIndex_r4/Relational  mode=a=b  en=off  latency=0  dbl_ovrd=off  block_type=relational
  sync_out : Outport
  valid_out : Outport  Port=2
  d_out : Outport  Port=3
  wires:
  Delay5/1 -> d_out/1  "d_out"
  Mux/1 -> valid_out/1  "valid"
  Constant1/1 -> Mux/2
  sync/1 -> chan_cnt/1, Delay1/1
  chan_cnt/1 -> chan_rel/1
  Slice2/1 -> chan_rel/2
  Constant2/1 -> Mux/3
  chan_rel/1 -> Mux/1
  chan_sel/1 -> Slice2/1, Slice/1
  Delay1/1 -> sync_out/1
  d_in0/1 -> Mux1/2
  d_in1/1 -> Mux1/3
  Mux1/1 -> Delay5/1
  Slice/1 -> Mux1/1
